simulink library "FaultInsertionUnit"  (Simulink 8.0)
settings: Solver=ode45  StartTime=0.0  StopTime=10.0  RelTol=1e-3
undefined symbols (not defined in the file): Ts
libraries: simulink x16
(part 2 of 2)

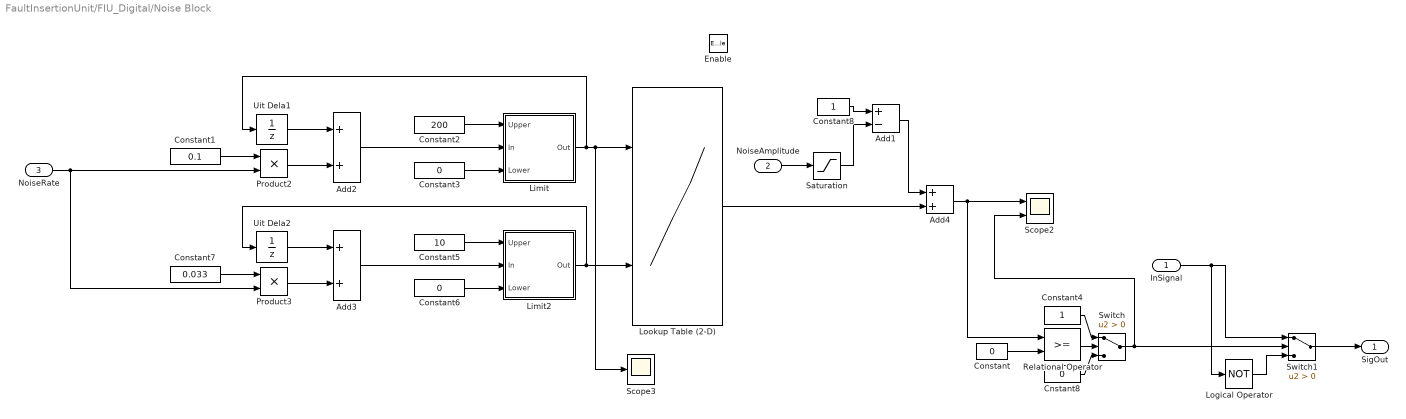
== system FaultInsertionUnit/FIU_Digital/Noise Block ==
  InSignal : Inport
  NoiseAmplitude : Inport  Port=2  OutDataTypeStr=double
  NoiseRate : Inport  Port=3
  Enable : EnablePort  StatesWhenEnabling=reset
  Add1 : Sum  Inputs=+-
  Add2 : Sum
  Add3 : Sum
  Add4 : Sum
  Cnstant8 : Constant  Value=0  OutDataTypeStr=double
  Constant : Constant  Value=0  OutDataTypeStr=double
  Constant1 : Constant  Value=0.1
  Constant2 : Constant  Value=200
  Constant3 : Constant  Value=0
  Constant4 : Constant  OutDataTypeStr=double
  Constant5 : Constant  Value=10
  Constant6 : Constant  Value=0
  Constant7 : Constant  Value=0.033
  Constant8 : Constant  OutDataTypeStr=double
  Limit : Subsystem
  Limit2 : Subsystem
  Logical Operator : Logic  Operator=NOT  AllPortsSameDT=off  OutDataTypeStr=boolean
  Lookup Table (2-D) : Lookup2D  RowIndex=[1:200]  ColumnIndex=[1:10]  Table=[0.059478 0.43661 -0.49306 0.23102 0.047775 0.32881 0.10527 -0.96761 -0.17936 -0.7715 ;-0.46458 -0.14226 -0.073569 -0.13391 -0.068713 -0.51372 -0.048223 -0.05778 -0.033297 -0.9336 ;0.69392 -0.63036 -0.42447 0.87456 0.21707 -0.02388 -0.10525 0.04543 0.19352 0.95965 ;-0.57043 -0.68679 0.90023 0.18436 0.88412 0.36409 -0.60649 0.27584 -0.46311 0.076011 ;0.51483 0.44455 -0.31639 0.44814 -0.79573 -0.91568 0.69359 0.52856 -0.51749 -0.27781 ;-0.46372 -0.7295 -0.58356 0.46135 0.76716 0.6258 -0.61754 0.45535 -0.73541 -0.86835 ;0.50488 0.74498 -0.20318 -0.26701 -0.2636 0.17345 0.55475 0.47207 -0.91499 -0.097736 ;-0.64441 -0.89804 0.34354 0.37527 0.28775 -0.9859 0.6495 -0.15923 0.78148 -0.35851 ;0.76434 -0.74859 -0.95771 -0.15581 0.81145 0.077942 -0.89502 -0.80833 -0.73444 -0.05261 ;-0.24648 -0.82401 -0.55611 0.8206 -0.20482 -0.47114 -0.56003 -0.71421 -0.43614 -0.6372 ;0.9408 0.91361 -0.0079724 -0.48861 0.19346 -0.086788 -0.76528 0.52495 -0.60627 0.0036683 ;0.47479 0.24439 0.82936 0.12246 -0.34564 0.88177 -0.29726 0.39259 -0.86418 0.6683 ;-0.010681 -0.4077 -0.080105 0.38061 0.47611 -0.82642 -0.39268 -0.039043 -0.086685 0.76899 ;0.65553 0.95958 -0.96498 -0.46645 -0.84307 0.9534 0.055539 0.30511 0.052539 0.57284 ;0.089641 0.83536 0.79567 -0.23709 -0.33065 0.29781 0.18052 -0.19083 0.37514 -0.0042971 ;-0.22126 0.58358 0.14929 0.12056 0.49933 -0.094293 0.65897 -0.58568 0.95792 0.80524 ;0.99764 -0.47973 -0.52224 0.74083 0.54483 -0.86987 0.16101 0.64042 0.6324 0.42208 ;0.33707 -0.4082 -0.75139 0.60465 -0.63416 0.39138 -0.21017 0.96892 -0.70009 -0.25507 ;0.0069244 -0.39533 -0.23039 -0.65718 -0.0096847 0.7163 0.51323 -0.43487 -0.26948 -0.85631 ;0.14176 0.85986 -0.44225 0.34414 0.44564 -0.13564 -0.93444 -0.38616 -0.28968 0.88197 ;-0.89037 -0.68029 0.6924 -0.63973 0.62656 -0.67392 -0.63956 -0.67534 0.76093 -0.96337 ;0.84891 -0.35158 -0.78584 -0.51018 -0.88655 -0.56286 0.89732 0.19436 0.53456 -0.10364 ;-0.90548 0.017171 0.71119 0.60675 -0.56683 -0.2331 -0.38058 0.44347 -0.33375 0.78087 ;0.5372 0.57766 0.21542 -0.048727 0.63165 0.41196 0.91552 -0.24646 -0.25985 0.1879 ;-0.64541 -0.89197 0.75662 0.92675 0.65934 0.10358 -0.67716 0.53513 -0.31431 -0.63993 ;0.64027 -0.45024 0.29231 0.19304 -0.94798 -0.07999 -0.31727 0.60419 -0.8408 0.62697 ;-0.60565 -0.3892 -0.11436 -0.69293 0.12092 0.9043 0.61038 0.51203 -0.45509 -0.68316 ;-0.18204 0.23803 -0.41733 0.89078 -0.7563 -0.42155 0.72326 -0.6621 -0.75891 0.63369 ;-0.43066 -0.78703 0.58854 -0.72774 -0.00028933 0.85117 0.6476 0.54839 -0.6327 0.37228 ;-0.52944 -0.63109 0.38573 -0.50185 0.44127 -0.27515 0.984 -0.47949 -0.34999 -0.25508 ;0.65462 -0.57956 0.64436 -0.55375 -0.0052001 0.56542 -0.49842 -0.39404 0.90475 -0.74693 ;-0.50147 0.63867 0.68479 -0.78925 -0.037871 -0.012363 -0.13535 0.86843 -0.92309 -0.35309 ;0.63539 0.75297 -0.066481 -0.39864 -0.77222 0.81742 0.84727 0.65968 -0.11524 0.69016 ;0.46389 0.74483 0.64082 0.70691 0.038276 0.44384 0.27706 -0.24474 0.79914 0.55669 ;0.34935 0.19564 -0.72728 0.34681 -0.0074384 -0.11379 -0.27504 -0.13171 0.60629 -0.46375 ;0.63704 -0.00029838 0.59022 -0.656 0.42108 0.6068 0.91679 -0.36743 -0.67755 0.45638 ;0.073564 0.5302 0.26019 0.53598 -0.63809 -0.36186 -0.76003 0.36121 -0.99579 0.2988 ;-0.65918 0.8818 -0.64919 -0.77877 -0.81473 -0.66233 -0.35199 0.54211 0.7532 0.21177 ;-0.30082 0.77817 0.27137 -0.59429 -0.80614 -0.5918 -0.53632 0.66567 -0.46164 -0.71729 ;-0.81883 -0.72359 -0.62828 -0.9465 -0.406 -0.17584 0.23429 0.86747 0.58099 -0.96536 ;0.54349 -0.31806 0.68759 0.35242 -0.1096 0.034494 0.62059 -0.86088 -0.51413 0.6079 ;-0.10989 -0.5256 -0.84164 0.4136 -0.93726 0.69895 -0.22816 -0.85528 0.058181 0.63288 ;-0.59386 -0.28897 0.55798 0.3372 0.43239 0.70489 0.12355 -0.5017 -0.41183 -0.31337 ;-0.028857 -0.43394 0.59069 0.35613 0.12777 -0.26627 0.63609 0.56775 0.13261 0.74048 ;0.28837 0.20258 -0.12991 0.4687 0.30789 0.90887 -0.15657 0.76172 -0.25952 0.39273 ;-0.66931 -0.59911 -0.077129 0.7496 -0.3623 0.99325 -0.64122 0.81862 -0.18906 0.10203 ;-0.94851 0.25736 0.79573 -0.96018 ...(+13218 chars) ]  LookUpMeth=Interpolation-Use End Values  OutDataTypeStr=double
  Product2 : Product  RndMeth=Zero
  Product3 : Product  RndMeth=Zero
  Relational Operator : RelationalOperator  OutDataTypeStr=boolean
  Saturation : Saturate  UpperLimit=1  LowerLimit=0
  Scope2 : Scope  NumInputPorts=2
      settings: YMin=-5~-5  YMax=5~5
  Scope3 : Scope
  Switch : Switch  Criteria=u2 > Threshold
  Switch1 : Switch  Criteria=u2 > Threshold
  Uit Dela1 : UnitDelay  SampleTime=-1
  Uit Dela2 : UnitDelay  SampleTime=-1
  SigOut : Outport
  wires:
  Uit Dela1/1 -> Add2/1
  Add2/1 -> Limit/2(In)
  Limit/1(Out) -> Uit Dela1/1, Lookup Table (2-D)/1, Scope3/1
  Constant2/1 -> Limit/1(Upper)
  Constant3/1 -> Limit/3(Lower)
  Uit Dela2/1 -> Add3/1
  Add3/1 -> Limit2/2(In)
  Limit2/1(Out) -> Uit Dela2/1, Lookup Table (2-D)/2
  Constant5/1 -> Limit2/1(Upper)
  Constant6/1 -> Limit2/3(Lower)
  Product2/1 -> Add2/2
  Constant1/1 -> Product2/1
  NoiseRate/1 -> Product2/2, Product3/2
  Product3/1 -> Add3/2
  Constant7/1 -> Product3/1
  Relational Operator/1 -> Switch/2
  Constant/1 -> Relational Operator/2
  Constant4/1 -> Switch/1
  Cnstant8/1 -> Switch/3
  Switch/1 -> Scope2/2, Switch1/2
  Add4/1 -> Scope2/1, Relational Operator/1
  Constant8/1 -> Add1/1
  NoiseAmplitude/1 -> Saturation/1
  Add1/1 -> Add4/1
  Saturation/1 -> Add1/2
  Lookup Table (2-D)/1 -> Add4/2
  InSignal/1 -> Switch1/1, Logical Operator/1
  Logical Operator/1 -> Switch1/3
  Switch1/1 -> SigOut/1

== system FaultInsertionUnit/FIU_Case/Delay Block/Subsystem ==
  DelayValueSet : Inport
  Constant : Constant  Value=Ts/2
  Relational Operator : RelationalOperator  Operator=<  OutDataTypeStr=boolean
  Relational Operator1 : RelationalOperator  Operator=>  OutDataTypeStr=boolean
  Sum : Sum  Inputs=|++
  Sum1 : Sum  Inputs=|+-
  Switch : Switch  Criteria=u2 > Threshold
  Switch2 : Switch  Criteria=u2 > Threshold
  Unit Delay : UnitDelay  SampleTime=-1
  DelayValueIs : Outport
  wires:
  Switch2/1 -> DelayValueIs/1, Unit Delay/1
  Sum1/1 -> Switch2/3
  Switch/1 -> Relational Operator1/2, Sum1/1, Switch2/1
  Relational Operator1/1 -> Switch2/2
  Constant/1 -> Sum1/2, Sum/2
  Sum/1 -> Switch/3
  Relational Operator/1 -> Switch/2
  Unit Delay/1 -> Relational Operator/2, Switch/1, Sum/1
  DelayValueSet/1 -> Relational Operator1/1, Relational Operator/1

== system FaultInsertionUnit/FIU_Countinuous/Delay Block/Subsystem ==
  DelayValueSet : Inport
  Ts : Inport  Port=2
  Gain : Gain  Gain=0.5
  Relational Operator : RelationalOperator  Operator=<  OutDataTypeStr=boolean
  Relational Operator1 : RelationalOperator  Operator=>  OutDataTypeStr=boolean
  Sum : Sum  Inputs=|++
  Sum1 : Sum  Inputs=|+-
  Switch : Switch  Criteria=u2 > Threshold
  Switch2 : Switch  Criteria=u2 > Threshold
  Unit Delay : UnitDelay  SampleTime=-1
  DelayValueIs : Outport
  wires:
  DelayValueSet/1 -> Relational Operator/1, Relational Operator1/1
  Unit Delay/1 -> Sum/1, Switch/1, Relational Operator/2
  Relational Operator/1 -> Switch/2
  Sum/1 -> Switch/3
  Gain/1 -> Sum/2, Sum1/2
  Relational Operator1/1 -> Switch2/2
  Switch/1 -> Switch2/1, Sum1/1, Relational Operator1/2
  Sum1/1 -> Switch2/3
  Switch2/1 -> Unit Delay/1, DelayValueIs/1
  Ts/1 -> Gain/1

== system FaultInsertionUnit/FIU_Countinuous/Noise Block/Limit ==
  Upper : Inport
  In : Inport  Port=2
  Lower : Inport  Port=3
  Relational Operator : RelationalOperator  Operator=<  OutDataTypeStr=boolean
  Subtract : Sum  Inputs=-+
  Subtract1 : Sum
  Switch : Switch
  Out : Outport
  wires:
  Lower/1 -> Subtract1/2
  Subtract/1 -> Subtract1/1
  Subtract1/1 -> Switch/1
  Switch/1 -> Out/1
  Relational Operator/1 -> Switch/2
  Upper/1 -> Subtract/1, Relational Operator/1
  In/1 -> Subtract/2, Switch/3, Relational Operator/2

== system FaultInsertionUnit/FIU_Countinuous/Noise Block/Limit2 ==
  Upper : Inport
  In : Inport  Port=2
  Lower : Inport  Port=3
  Relational Operator : RelationalOperator  Operator=<  OutDataTypeStr=boolean
  Subtract : Sum  Inputs=-+
  Subtract1 : Sum
  Switch : Switch
  Out : Outport
  wires:
  In/1 -> Relational Operator/2, Switch/3, Subtract/2
  Upper/1 -> Relational Operator/1, Subtract/1
  Relational Operator/1 -> Switch/2
  Switch/1 -> Out/1
  Subtract1/1 -> Switch/1
  Subtract/1 -> Subtract1/1
  Lower/1 -> Subtract1/2

== system FaultInsertionUnit/FIU_Countinuous/Slewrate Block/ArbitrateSignalChange ==
  RequestedSignalChange : Inport
  SlewRate : Inport  Port=2
  SamplingTime : Inport  Port=3
  Abs : Abs
  Divide : Product  Inputs=**
  Gain : Gain
  Gain1 : Gain  Gain=-1
  Limit : Subsystem
  AcceptedSignalChange : Outport
  wires:
  Gain1/1 -> Limit/3(Lower)
  Gain/1 -> Limit/1(Upper)
  Limit/1(Out) -> AcceptedSignalChange/1
  RequestedSignalChange/1 -> Limit/2(In)
  Abs/1 -> Divide/1
  Divide/1 -> Gain1/1, Gain/1  "MaxChangePerCycle"
  SamplingTime/1 -> Divide/2
  SlewRate/1 -> Abs/1

== system FaultInsertionUnit/FIU_Digital/Delay Block/Subsystem ==
  DelayValueSet : Inport
  Constant : Constant  Value=Ts/2
  Relational Operator : RelationalOperator  Operator=<  OutDataTypeStr=boolean
  Relational Operator1 : RelationalOperator  Operator=>  OutDataTypeStr=boolean
  Sum : Sum  Inputs=|++
  Sum1 : Sum  Inputs=|+-
  Switch : Switch  Criteria=u2 > Threshold
  Switch2 : Switch  Criteria=u2 > Threshold
  Unit Delay : UnitDelay  SampleTime=-1
  DelayValueIs : Outport
  wires:
  Switch2/1 -> DelayValueIs/1, Unit Delay/1
  Sum1/1 -> Switch2/3
  Switch/1 -> Relational Operator1/2, Sum1/1, Switch2/1
  Relational Operator1/1 -> Switch2/2
  Constant/1 -> Sum1/2, Sum/2
  Sum/1 -> Switch/3
  Relational Operator/1 -> Switch/2
  Unit Delay/1 -> Relational Operator/2, Switch/1, Sum/1
  DelayValueSet/1 -> Relational Operator1/1, Relational Operator/1

== system FaultInsertionUnit/FIU_Digital/Noise Block/Limit ==
  Upper : Inport
  In : Inport  Port=2
  Lower : Inport  Port=3
  Relational Operator : RelationalOperator  Operator=<  OutDataTypeStr=boolean
  Subtract : Sum  Inputs=-+
  Subtract1 : Sum
  Switch : Switch
  Out : Outport
  wires:
  Lower/1 -> Subtract1/2
  Subtract/1 -> Subtract1/1
  Subtract1/1 -> Switch/1
  Switch/1 -> Out/1
  Relational Operator/1 -> Switch/2
  Upper/1 -> Subtract/1, Relational Operator/1
  In/1 -> Subtract/2, Switch/3, Relational Operator/2

== system FaultInsertionUnit/FIU_Digital/Noise Block/Limit2 ==
  Upper : Inport
  In : Inport  Port=2
  Lower : Inport  Port=3
  Relational Operator : RelationalOperator  Operator=<  OutDataTypeStr=boolean
  Subtract : Sum  Inputs=-+
  Subtract1 : Sum
  Switch : Switch
  Out : Outport
  wires:
  In/1 -> Relational Operator/2, Switch/3, Subtract/2
  Upper/1 -> Relational Operator/1, Subtract/1
  Relational Operator/1 -> Switch/2
  Switch/1 -> Out/1
  Subtract1/1 -> Switch/1
  Subtract/1 -> Subtract1/1
  Lower/1 -> Subtract1/2

== system FaultInsertionUnit/FIU_Countinuous/Slewrate Block/ArbitrateSignalChange/Limit ==
  Upper : Inport
  In : Inport  Port=2
  Lower : Inport  Port=3
  MinMax : MinMax  Inputs=2
  MinMax1 : MinMax  Function=max  Inputs=2
  Out : Outport
  wires:
  MinMax1/1 -> Out/1
  Lower/1 -> MinMax1/2
  MinMax/1 -> MinMax1/1
  Upper/1 -> MinMax/1
  In/1 -> MinMax/2
